simulink model "MovingObject"  (Simulink 7.6)
settings: Solver=FixedStepDiscrete  StartTime=0.0  StopTime=inf  RelTol=1e-3
model workspace: external: M-Code (data not in the file)
undefined symbols (not defined in the file): gray, Rec, SDTV
libraries: vipconversions x2, viptextngfix x1, dspsrcs4 x1, vipstatistics x1, vipsnks x1
CloseFcn:
  | clear line_row;
settings Model: Creator=don  LastModifiedBy=hzarrink  ExtModeAutoUpdateStatusClock=off
settings DataIOCC: LimitDataPoints=off  SaveOutput=off  SignalLogging=off  SaveTime=off  SignalLoggingName=sigsOut
settings OptimizationCC: InitFltsAndDblsToZero=on  EfficientMapNaN2IntZero=off  BufferReusableBoundary=off
settings DebuggingCC: AlgebraicLoopMsg=none  SaveWithParameterizedLinksMsg=none  CheckExecutionContextPreStartOutputMsg=on  CheckExecutionContextRuntimeOutputMsg=on  SignalResolutionControl=TryResolveAllWithWarning  SolverPrmCheckMsg=none  MultiTaskDSMMsg=warning  MultiTaskCondExecSysMsg=none  ParameterPrecisionLossMsg=none  BusObjectLabelMismatch=none  StrictBusMsg=None
settings HardwareCC: TargetHWDeviceType=32-bit Generic  ProdEqTarget=off
settings SFSimCC: SimParseCustomCode=off
settings RTWCC: IncludeERTFirstTime=on
settings GRTTargetCC: TargetFcnLib=ansi_tfl_tmw.mat

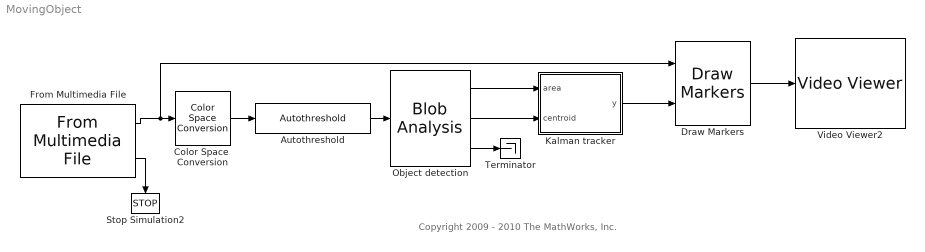
== system MovingObject ==
  note: Copyright 2009 - 2010 The MathWorks, Inc.
  Autothreshold : vipconversions/Autothreshold  DialogController=vipDDGCreate  DialogControllerArgs=DataTag0  operator=<=  threshOut=off  effMetricOut=off  userDefinedRange=off  umin=0  umax=255  outOfRngOpt=Warn and saturate  scaleThreshold=off  scaleFactor=1  P1Mode=Specify word length  P1WordLength=32  P1FracLength=30  P2Mode=Specify word length  P2WordLength=32  P2FracLength=22  P3Mode=Specify word length  P3WordLength=32  P3FracLength=14  P4Mode=Binary point scaling  P4WordLength=32  P4FracLength=15  Q1Mode=Specify word length  Q1WordLength=32  Q1FracLength=16  EMMode=Specify word length  EMWordLength=16  EMFracLength=14  roundingMode=Floor  overflowMode=off
  Color Space  Conversion : vipconversions/Color Space  Conversion  conversion=Obsolete  conversionActive=R'G'B' to intensity  wp_str=D65  rec=Rec. 601 (SDTV)  sys=1125/60/2:1  imagePorts=One multidimensional signal
  Draw Markers : viptextngfix/Draw Markers  DialogController=vipDDGCreate  DialogControllerArgs=DataTag1  shape=X-mark  size=10  fill=off  fillClrSource=Specify via dialog  display=User-specified value  intensity=200  color=[255 0 0]  opacity=0.6  viewport=Entire image  antialiasing=off  inType=Obsolete  imagePorts=One multidimensional signal  prodOutputMode=Binary point scaling  prodOutputWordLength=32  prodOutputFracLength=14  memoryMode=Specify word length  memoryWordLength=16  memoryFracLength=15  roundingMode=Floor  overflowMode=off
  From Multimedia File : dspsrcs4/From Multimedia File  DialogController=dspDDGCreate  DialogControllerArgs=DataTag2  inputFilename=MovingObject.avi  loop=on  numPlays=1  outputStreams=Video only  videoDataType=double  audioDataType=int16  inheritSampleTime=on  userDefinedSampleTime=1/40  noAudioOutput=off  isIntensityVideo=off  fourcc=RGB  colorVideoFormat=One multidimensional signal  outputEOF=on  dataOrg=Column-major  audioFrameSize=1024  computeAudioFrameSize=off
  Kalman tracker : Stateflow chart  TreatAsAtomicUnit=on
  Object detection : vipstatistics/Blob Analysis  Tag=vipblks_row_conv  DialogController=vipDDGCreate  DialogControllerArgs=DataTag3  area=on  centroid=on  bBox=off  majorAxis=off  minorAxis=off  angle=off  eccentricity=off  equivDiameterSq=off  extent=off  perimeter=off  maxBlobs=20  warnIfNumBlobsExceeded=off  isCount=on  useMinArea=on  minArea=1  useMaxArea=on  maxArea=100000  excludeBorderBlob=off  outDT=double  isOutVarDim=off  isFill=on  fillValues=0  conn=8  isLabel=off  outputMode=Binary point scaling  outputWordLength=32  outputFracLength=16  firstCoeffMode=Binary point scaling  firstCoeffWordLength=16  firstCoeffFracLength=14  secondCoeffMode=Binary point scaling  secondCoeffWordLength=32  secondCoeffFracLength=16  accumMode=Binary point scaling  accumWordLength=32  accumFracLength=0  prodOutputMode=Binary point scaling  prodOutputWordLength=32  prodOutputFracLength=16  roundingMode=Zero  overflowMode=off
  Stop Simulation2 : Stop
  Terminator : Terminator
  Video Viewer2 : vipsnks/Video Viewer  DialogControllerArgs=DataTag5  inputType=Obsolete7b  imagePorts=One multidimensional signal  useColorMap=off  colormapValue=gray(256)  specRange=off  minInputVal=0  maxInputVal=255  FigPos=[670 712 338 225]  AxisZoom=on  trueSizedOnce=off  OpenAtMdlStart=on
  wires:
  Autothreshold/1 -> Object detection/1
  Object detection/1 -> Kalman tracker/1(area)
  Draw Markers/1 -> Video Viewer2/1
  Object detection/2 -> Kalman tracker/2(centroid)
  From Multimedia File/2 -> Stop Simulation2/1
  Kalman tracker/1(y) -> Draw Markers/2
  Color Space  Conversion/1 -> Autothreshold/1
  From Multimedia File/1 -> Color Space  Conversion/1, Draw Markers/1
  Object detection/3 -> Terminator/1

== matlab function Kalman tracker ==
  data: area input double; y output double; centroid input double
function y = kalman(area,centroid)
%#eml
[v,i]=max(area);
z=centroid(:,i);
y=kalman01(z);
